simulink model "HW7_v2_simulink"  (R2019b)
settings: Solver=VariableStepAuto  StartTime=0.0  StopTime=15  RelTol=1e-3
values from neighbouring files (symbols this model uses):
  A = double(round(subs(J_x,   [states, inputs], [trim_state, trim_input])*1000)/1000)    [state_decoupling.m]
  A1_wiener = [0 1 ;               0 0]    [HW7_v2_matlab.m]
  Aaileron = A(5:8,5:8)    [state_decoupling.m]
  Aelevator = A(1:4,1:4)    [state_decoupling.m]
  Arudder = A(11:12,11:12)    [state_decoupling.m]
  Athrust = A(9:10,9:10)    [state_decoupling.m]
  B = B*MotorMix    [state_decoupling.m]
  B1_wiener = [0;               1]    [HW7_v2_matlab.m]
  Baileron = B(5:8,3)    [state_decoupling.m]
  Belevator = B(1:4,2)    [state_decoupling.m]
  Brudder = B(11:12,4)    [state_decoupling.m]
  Bthrust = B(9:10,1)    [state_decoupling.m]
  C = double(round(subs(J_y,   [states, inputs], [trim_state, trim_input])*1000)/1000)    [state_decoupling.m]
  C1_wiener = [1 0]    [HW7_v2_matlab.m]
  C_P = 0.041    [state_decoupling.m]
  C_rollpitch = rho*prop_dia^4*prop_dist/sqrt(2)*[                 1  -1  -1   1 ;                 1   1  -1  -1 ;                 0   0   0   0 ; ]    [state_decoupling.m]
  C_T = [0.069075;4.95e-05]    [state_decoupling.m]
  C_yaw = rho*prop_dia^5/(2*pi)*[                 0   0   0   0 ;                 0   0   0   0 ;                -1   1  -1   1 ; ]    [state_decoupling.m]
  Caileron = [0 1 0 0; 0 0 0 1]    [state_decoupling.m]
  Celevator = [0 1 0 0; 0 0 0 1]    [state_decoupling.m]
  Crudder = [0 1]    [state_decoupling.m]
  Cthrust = [ 1 0; 0 0]    [state_decoupling.m]
  D = D*MotorMix    [state_decoupling.m]
  D1_wiener = [0]    [HW7_v2_matlab.m]
  Daileron = [0 ; 0]    [state_decoupling.m]
  Delevator = [0 ; 0]    [state_decoupling.m]
  Drudder = 0    [state_decoupling.m]
  Dthrust = [0 ; D(4,1)]    [state_decoupling.m]
  g = [0;0;UAV_mass*9.81]    [state_decoupling.m]
  J = [      Jxx   0   0 ;       0   Jyy  0 ;       0    0  Jzz; ]    [state_decoupling.m]
  Jinv = inv(J)    [state_decoupling.m]
  Kaileron = Kaileron(2:4)    [HW7_v2_matlab.m]
  Kelevator = Kelevator(2:4)    [HW7_v2_matlab.m]
  Krudder = Krudder(2)    [HW7_v2_matlab.m]
  Kthrust = lqr(Athrust, Bthrust, Qthrust, Rthrust)    [HW7_v2_matlab.m]
  L1 = lqe(A1_cont, G1, C1_cont, Q1, R1, N1)    [HW7_v2_matlab.m]
  M_inv = inv(M_motor)    [HW7_v2_matlab.m]
  M_motor = [1, 1, 1, -1;             1, 1, -1, 1;             1, -1, -1, -1;             1, -1, 1, 1 ]    [HW7_v2_matlab.m]
  Prop_H = 2*pi*Jprop*[               0  0  0  0 ;               0  0  0  0 ;               1 -1  1 -1 ; ]    [state_decoupling.m]
  tau2 = eval(max(solve(1/sqrt((tau2*2*pi*10)^2+1^2) == 1/sqrt(2), tau2)))    [HW7_v2_matlab.m]
  Thrust_Sum = rho*prop_dia^4*[                 0   0   0   0 ;                 0   0   0   0 ;                -1  -1  -1  -1 ; ]    [state_decoupling.m]
  trim_state = [0,0,0,0,0,0,0,0,0,0,0,0]    [state_decoupling.m]
  UAV_mass = 0.068    [state_decoupling.m]
undefined symbols (not defined in the file or in its folder): DiscIntNeverNeededParam, measurement_noise
libraries: simulink x5, vrlib x3, dspmtrx3 x1
settings Model: Creator=cwhipp  LastModifiedBy=cwhipp

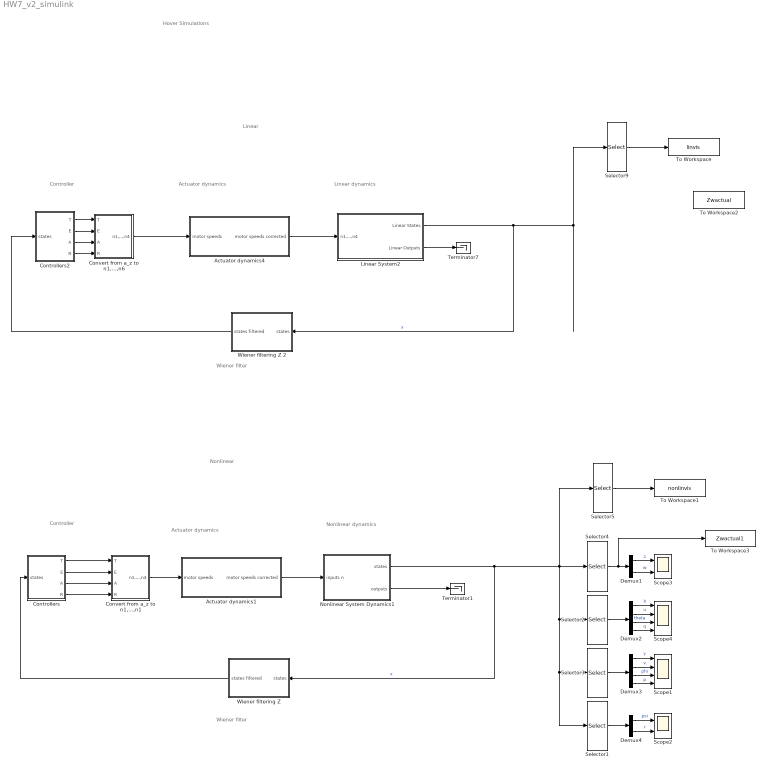
== system HW7_v2_simulink ==
  note: Hover Simulations
  note: Nonlinear
  note: Linear
  note: Controller
  note: Actuator dynamics
  note: Linear dynamics
  note: Wiener filter
  note: Controller
  note: Actuator dynamics
  note: Nonlinear dynamics
  note: Wiener filter
  Actuator dynamics1 : Subsystem
  Actuator dynamics4 : Subsystem
  Controllers : Subsystem
  Controllers2 : Subsystem
  Convert from a_z to n1,...,n1 : Subsystem
  Convert from a_z to n1,...,n6 : Subsystem
  Demux1 : Demux  Outputs=2
  Demux2 : Demux
  Demux3 : Demux
  Demux4 : Demux  Outputs=2
  Linear System2 : Subsystem
  Nonlinear System Dynamics1 : Subsystem
  Scope1 : Scope  NumInputPorts=4
  Scope2 : Scope  NumInputPorts=2
  Scope3 : Scope  NumInputPorts=2
  Scope4 : Scope  NumInputPorts=4
  Selector1 : Selector  InputPortWidth=12  IndexOptions=Index vector (dialog)  Indices=[11 12]  OutputSizes=1
  Selector2 : Selector  InputPortWidth=12  IndexOptions=Index vector (dialog)  Indices=[3 4 5 6]  OutputSizes=1
  Selector3 : Selector  InputPortWidth=12  IndexOptions=Index vector (dialog)  Indices=[7 8 9 10]  OutputSizes=1
  Selector4 : Selector  InputPortWidth=12  IndexOptions=Index vector (dialog)  Indices=[1 2]  OutputSizes=1
  Selector5 : Selector  InputPortWidth=12  IndexOptions=Index vector (dialog)  Indices=[3 7 1 5 9 11]  OutputSizes=1
  Selector9 : Selector  InputPortWidth=12  IndexOptions=Index vector (dialog)  Indices=[3 7 1 5 9 11]  OutputSizes=1
  Terminator1 : Terminator
  Terminator7 : Terminator
  To Workspace : ToWorkspace  VariableName=linvis  SampleTime=-1
      settings: Save2DSignal=2-D array (concatenate along first dimension)
  To Workspace1 : ToWorkspace  VariableName=nonlinvis  SampleTime=-1
      settings: Save2DSignal=2-D array (concatenate along first dimension)
  To Workspace2 : ToWorkspace  VariableName=Zwactual  SaveFormat=Timeseries  SampleTime=-1
  To Workspace3 : ToWorkspace  VariableName=Zwactual1  SaveFormat=Timeseries  SampleTime=-1
  "Wiener filtering Z " : Subsystem
  Wiener filtering Z 2 : Subsystem
  wires:
  Actuator dynamics1/1(motor speeds corrected) -> Nonlinear System Dynamics1/1(inputs n)
  Controllers/4(R) -> Convert from a_z to n1,...,n1/4(R)
  Convert from a_z to n1,...,n1/1(n1,...,n4) -> Actuator dynamics1/1(motor speeds)
  Nonlinear System Dynamics1/2(outputs) -> Terminator1/1
  Controllers/3(A) -> Convert from a_z to n1,...,n1/3(A)
  "Wiener filtering Z "/1("states filtered ") -> Controllers/1(states)
  Controllers/1(T) -> Convert from a_z to n1,...,n1/1(T)
  Controllers/2(E) -> Convert from a_z to n1,...,n1/2(E)
  Actuator dynamics4/1(motor speeds corrected) -> Linear System2/1(n1,...,n4)
  Controllers2/1(T) -> Convert from a_z to n1,...,n6/1(T)
  Convert from a_z to n1,...,n6/1(n1,...,n4) -> Actuator dynamics4/1(motor speeds)
  Controllers2/2(E) -> Convert from a_z to n1,...,n6/2(E)
  Controllers2/4(R) -> Convert from a_z to n1,...,n6/4(R)
  Wiener filtering Z 2/1("states filtered ") -> Controllers2/1(states)
  Controllers2/3(A) -> Convert from a_z to n1,...,n6/3(A)
  Linear System2/2(Linear Outputs) -> Terminator7/1
  Demux4/2 -> Scope2/2  "r"
  Demux3/1 -> Scope1/1  "Y"
  Demux1/1 -> Scope3/1  "z"
  Demux2/4 -> Scope4/4  "q"
  Demux2/3 -> Scope4/3  "theta"
  Demux4/1 -> Scope2/1  "psi"
  Demux2/2 -> Scope4/2  "u"
  Demux1/2 -> Scope3/2  "w"
  Demux3/3 -> Scope1/3  "phi"
  Selector3/1 -> Demux3/1
  Demux2/1 -> Scope4/1  "X"
  Selector1/1 -> Demux4/1
  Selector4/1 -> To Workspace3/1, Demux1/1
  Demux3/4 -> Scope1/4  "p"
  Nonlinear System Dynamics1/1(states) -> Selector5/1, Selector1/1, Selector3/1, Selector2/1, Selector4/1, "Wiener filtering Z "/1(states)  "x"
  Selector2/1 -> Demux2/1
  Demux3/2 -> Scope1/2  "v"
  Selector9/1 -> To Workspace/1
  Linear System2/1(Linear States) -> Selector9/1, Wiener filtering Z 2/1(states)  "x"
  Selector5/1 -> To Workspace1/1

== system HW7_v2_simulink/Actuator dynamics1 ==
  motor speeds : Inport
  30ms delay : TransportDelay  DelayTime=30e-3
  Demux : Demux
  Mux : Mux
  Saturation4 : Saturate  UpperLimit=500  LowerLimit=10
  Sum2 : Sum  Inputs=++|
  Transfer Fcn : TransferFcn  Denominator=[tau2 1]
  Transfer Fcn1 : TransferFcn  Denominator=[tau2 1]
  Transfer Fcn2 : TransferFcn  Denominator=[tau2 1]
  actuator transfer function : TransferFcn  Denominator=[tau2 1]
  speed correction : Constant  Value=293
  motor speeds corrected : Outport
  wires:
  speed correction/1 -> Sum2/1
  Sum2/1 -> Saturation4/1
  Demux/2 -> Transfer Fcn1/1
  30ms delay/1 -> Demux/1
  Demux/4 -> actuator transfer function/1
  Demux/1 -> Transfer Fcn/1
  Demux/3 -> Transfer Fcn2/1
  Transfer Fcn/1 -> Mux/1
  Transfer Fcn1/1 -> Mux/2
  Transfer Fcn2/1 -> Mux/3
  actuator transfer function/1 -> Mux/4
  Mux/1 -> Sum2/2
  Saturation4/1 -> motor speeds corrected/1
  motor speeds/1 -> 30ms delay/1

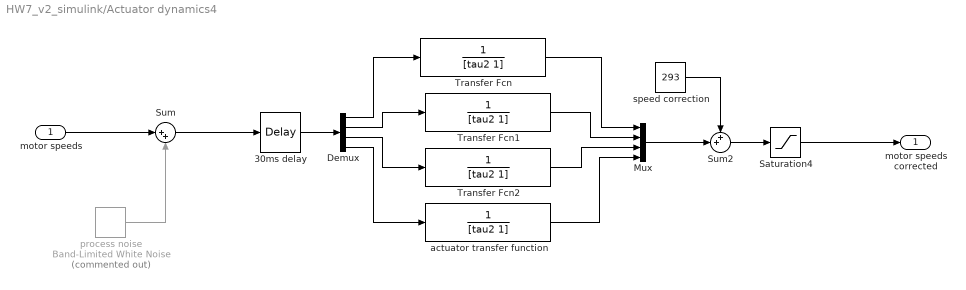
== system HW7_v2_simulink/Actuator dynamics4 ==
  motor speeds : Inport
  30ms delay : TransportDelay  DelayTime=30e-3
  Demux : Demux
  Mux : Mux
  Saturation4 : Saturate  UpperLimit=500  LowerLimit=10
  Sum : Sum  Inputs=|++
  Sum2 : Sum  Inputs=++|
  Transfer Fcn : TransferFcn  Denominator=[tau2 1]
  Transfer Fcn1 : TransferFcn  Denominator=[tau2 1]
  Transfer Fcn2 : TransferFcn  Denominator=[tau2 1]
  actuator transfer function : TransferFcn  Denominator=[tau2 1]
  process noise : simulink/Sources/Band-Limited White Noise  Commented=on  Cov=0.005*[1; 1; 1; 1]  Ts=0.005  seed=[1; 2; 3; 4]
  speed correction : Constant  Value=293  SampleTime=0.005
  motor speeds corrected : Outport
  wires:
  speed correction/1 -> Sum2/1
  Sum2/1 -> Saturation4/1
  Demux/2 -> Transfer Fcn1/1
  30ms delay/1 -> Demux/1
  Demux/4 -> actuator transfer function/1
  Demux/1 -> Transfer Fcn/1
  Demux/3 -> Transfer Fcn2/1
  Transfer Fcn/1 -> Mux/1
  Transfer Fcn1/1 -> Mux/2
  Transfer Fcn2/1 -> Mux/3
  actuator transfer function/1 -> Mux/4
  Mux/1 -> Sum2/2
  Saturation4/1 -> motor speeds corrected/1
  process noise/1 -> Sum/2
  motor speeds/1 -> Sum/1
  Sum/1 -> 30ms delay/1

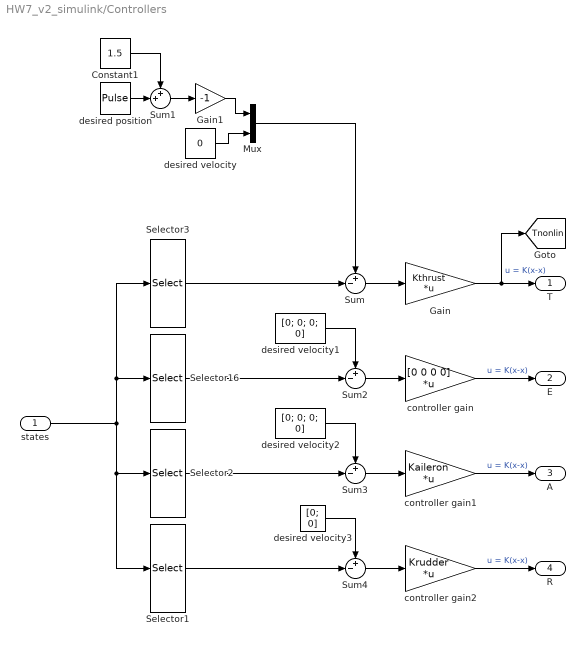
== system HW7_v2_simulink/Controllers ==
  states : Inport
  Constant1 : Constant  Value=1.5  SampleTime=0.05
  Gain : Gain  Gain=Kthrust  Multiplication=Matrix(K*u)
  Gain1 : Gain  Gain=-1
  Mux : Mux  Inputs=2
  Selector1 : Selector  InputPortWidth=12  IndexOptions=Index vector (dialog)  Indices=[11 12]  OutputSizes=1
  Selector16 : Selector  InputPortWidth=12  IndexOptions=Index vector (dialog)  Indices=[3 4 5 6]  OutputSizes=1
  Selector2 : Selector  InputPortWidth=12  IndexOptions=Index vector (dialog)  Indices=[7 8 9 10]  OutputSizes=1
  Selector3 : Selector  InputPortWidth=12  IndexOptions=Index vector (dialog)  Indices=[1 2]  OutputSizes=1
  Sum{,2..4} (4 alike) : Sum  Inputs=+-|
  Sum1 : Sum  Inputs=++|
  controller gain : Gain  Gain=[0 0 0 0]  Multiplication=Matrix(K*u)
  controller gain1 : Gain  Gain=Kaileron  Multiplication=Matrix(K*u)
  controller gain2 : Gain  Gain=Krudder  Multiplication=Matrix(K*u)
  desired position : DiscretePulseGenerator  PulseType=Time based  Amplitude=-1.5  Period=10  PulseWidth=50
  desired velocity : Constant  Value=0  SampleTime=0.05
  desired velocity1 : Constant  Value=[0; 0; 0; 0]  SampleTime=0.05
  desired velocity2 : Constant  Value=[0; 0; 0; 0]  SampleTime=0.05
  desired velocity3 : Constant  Value=[0; 0]  SampleTime=0.05
  T : Outport
  E : Outport  Port=2
  A : Outport  Port=3
  R : Outport  Port=4
  tag scope: Tnonlin=global
  wires:
  states/1 -> Selector16/1, Selector3/1, Selector1/1, Selector2/1
  Mux/1 -> Sum/1
  Gain1/1 -> Mux/1
  Sum/1 -> Gain/1
  Sum1/1 -> Gain1/1
  Selector3/1 -> Sum/2
  Constant1/1 -> Sum1/1
  Gain/1 -> [Tnonlin], T/1  "u = K(x-x)"
  desired position/1 -> Sum1/2
  Selector16/1 -> Sum2/2
  desired velocity1/1 -> Sum2/1
  Sum2/1 -> controller gain/1
  controller gain/1 -> E/1  "u = K(x-x)"
  Selector2/1 -> Sum3/2
  controller gain1/1 -> A/1  "u = K(x-x)"
  desired velocity2/1 -> Sum3/1
  Sum3/1 -> controller gain1/1
  controller gain2/1 -> R/1  "u = K(x-x)"
  Sum4/1 -> controller gain2/1
  desired velocity3/1 -> Sum4/1
  Selector1/1 -> Sum4/2
  desired velocity/1 -> Mux/2

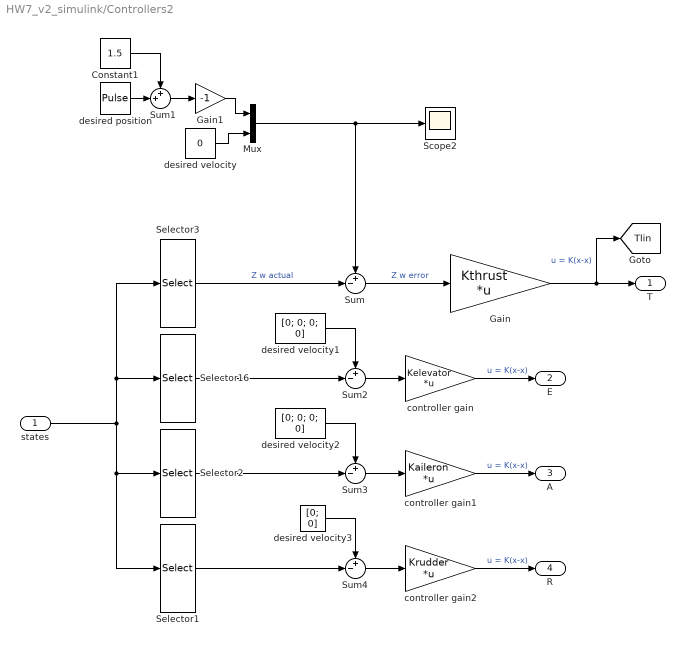
== system HW7_v2_simulink/Controllers2 ==
  states : Inport
  Constant1 : Constant  Value=1.5  SampleTime=0.05
  Gain : Gain  Gain=Kthrust  Multiplication=Matrix(K*u)
  Gain1 : Gain  Gain=-1
  Mux : Mux  Inputs=2
  Scope2 : Scope
  Selector1 : Selector  InputPortWidth=12  IndexOptions=Index vector (dialog)  Indices=[11 12]  OutputSizes=1
  Selector16 : Selector  InputPortWidth=12  IndexOptions=Index vector (dialog)  Indices=[3 4 5 6]  OutputSizes=1
  Selector2 : Selector  InputPortWidth=12  IndexOptions=Index vector (dialog)  Indices=[7 8 9 10]  OutputSizes=1
  Selector3 : Selector  InputPortWidth=12  IndexOptions=Index vector (dialog)  Indices=[1 2]  OutputSizes=1
  Sum{,2..4} (4 alike) : Sum  Inputs=+-|
  Sum1 : Sum  Inputs=++|
  controller gain : Gain  Gain=Kelevator  Multiplication=Matrix(K*u)
  controller gain1 : Gain  Gain=Kaileron  Multiplication=Matrix(K*u)
  controller gain2 : Gain  Gain=Krudder  Multiplication=Matrix(K*u)
  desired position : DiscretePulseGenerator  PulseType=Time based  Amplitude=-1.5  Period=10  PulseWidth=50
  desired velocity : Constant  Value=0  SampleTime=0.05
  desired velocity1 : Constant  Value=[0; 0; 0; 0]  SampleTime=0.05
  desired velocity2 : Constant  Value=[0; 0; 0; 0]  SampleTime=0.05
  desired velocity3 : Constant  Value=[0; 0]  SampleTime=0.05
  T : Outport
  E : Outport  Port=2
  A : Outport  Port=3
  R : Outport  Port=4
  tag scope: Tlin=global
  wires:
  states/1 -> Selector16/1, Selector3/1, Selector2/1, Selector1/1
  Mux/1 -> Scope2/1, Sum/1
  Gain1/1 -> Mux/1
  Sum/1 -> Gain/1  "Z w error"
  Sum1/1 -> Gain1/1
  Constant1/1 -> Sum1/1
  Gain/1 -> T/1, [Tlin]  "u = K(x-x)"
  desired position/1 -> Sum1/2
  desired velocity1/1 -> Sum2/1
  Sum2/1 -> controller gain/1
  controller gain/1 -> E/1  "u = K(x-x)"
  controller gain1/1 -> A/1  "u = K(x-x)"
  desired velocity2/1 -> Sum3/1
  Sum3/1 -> controller gain1/1
  controller gain2/1 -> R/1  "u = K(x-x)"
  Sum4/1 -> controller gain2/1
  desired velocity3/1 -> Sum4/1
  desired velocity/1 -> Mux/2
  Selector3/1 -> Sum/2  "Z w actual"
  Selector16/1 -> Sum2/2
  Selector2/1 -> Sum3/2
  Selector1/1 -> Sum4/2

== system HW7_v2_simulink/Convert from a_z to n1,...,n1 ==
  T : Inport
  E : Inport  Port=2
  A : Inport  Port=3
  R : Inport  Port=4
  Convert fom TEAR to n1,..,n4 : Gain  Gain=M_motor  Multiplication=Matrix(K*u)
  Mux : Mux
  n1,...,n4 : Outport
  wires:
  Convert fom TEAR to n1,..,n4/1 -> n1,...,n4/1
  Mux/1 -> Convert fom TEAR to n1,..,n4/1
  T/1 -> Mux/1
  E/1 -> Mux/2
  A/1 -> Mux/3
  R/1 -> Mux/4

== system HW7_v2_simulink/Convert from a_z to n1,...,n6 ==
  T : Inport
  E : Inport  Port=2
  A : Inport  Port=3
  R : Inport  Port=4
  Convert fom TEAR to n1,..,n4 : Gain  Gain=M_motor  Multiplication=Matrix(K*u)
  Mux : Mux
  n1,...,n4 : Outport
  wires:
  Convert fom TEAR to n1,..,n4/1 -> n1,...,n4/1
  Mux/1 -> Convert fom TEAR to n1,..,n4/1
  T/1 -> Mux/1
  E/1 -> Mux/2
  A/1 -> Mux/3
  R/1 -> Mux/4

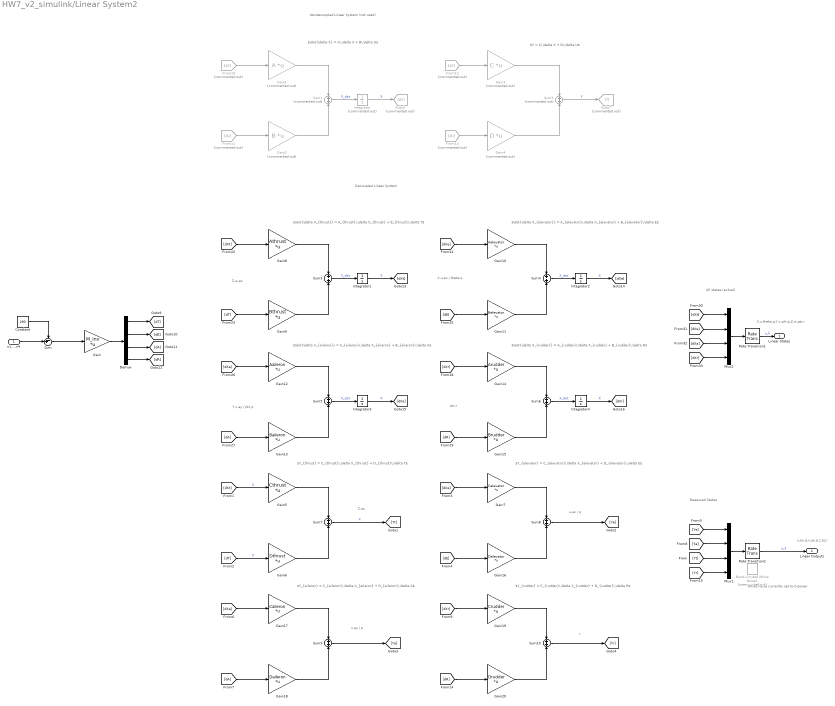
== system HW7_v2_simulink/Linear System2 ==
  note: psi,r
  note: Y,v,ay / phi,p
  note: X,u,ax / theta,q
  note: Z,w,az
  note: Decoupled Linear System
  note: $\dot{\delta X} = A\,\delta X + B\,\delta U$
  note: $Y = C\,\delta X + D\,\delta U$
  note: $\dot{\delta X_{thrust}} = A_{thrust}\,\delta X_{thrust} + B_{thrust}\,\delta T$
  note: $\dot{\delta X_{elevator}} = A_{elevator}\,\delta X_{elevator} + B_{elevator}\,\delta E$
  note: $\dot{\delta X_{aileron}} = A_{aileron}\,\delta X_{aileron} + B_{aileron}\,\delta A$
  note: $\dot{\delta X_{rudder}} = A_{rudder}\,\delta X_{rudder} + B_{rudder}\,\delta R$
  note: Z,az
  note: u,ax / q
  note: v,ay / p
  note: r
  note: $Y_{thrust} = C_{thrust}\,\delta X_{thrust} + D_{thrust}\,\delta T$
  note: $Y_{elevator} = C_{elevator}\,\delta X_{elevator} + D_{elevator}\,\delta E$
  note: $Y_{aileron} = C_{aileron}\,\delta X_{aileron} + D_{aileron}\,\delta A$
  note: $Y_{rudder} = C_{rudder}\,\delta X_{rudder} + D_{rudder}\,\delta R$
  note: Nondecoupled Linear System (not used)
  note: All states (actual)
  note: Measured States
  note: u,ax,q,v,ay,p,z,az,r
  note: X,u,theta,q,Y,v,phi,p,Z,w,psi,r
  note: White noise currently set to 0 power
  n1,...,n4 : Inport
  Band-Limited White Noise1 : simulink/Sources/Band-Limited White Noise  Commented=on  Cov=measurement_noise*ones(9,1)*0  Ts=0.05  seed=[11;12;13;14;15;16;17;18;19]
  Constant : Constant  Value=293
  Demux : Demux
  From10 : From  Commented=on  GotoTag=dX
  From11 : From  Commented=on  GotoTag=dU
  From12 : From  Commented=on  GotoTag=dX
  From13 : From  Commented=on  GotoTag=dU
  Gain : Gain  Gain=M_inv  Multiplication=Matrix(K*u)
  Gain1 : Gain  Commented=on  Gain=A  Multiplication=Matrix(K*u)
  Gain10 : Gain  Gain=Aelevator  Multiplication=Matrix(K*u)
  Gain11 : Gain  Gain=Belevator  Multiplication=Matrix(K*u)
  Gain12 : Gain  Gain=Aaileron  Multiplication=Matrix(K*u)
  Gain13 : Gain  Gain=Baileron  Multiplication=Matrix(K*u)
  Gain14 : Gain  Gain=Arudder  Multiplication=Matrix(K*u)
  Gain15 : Gain  Gain=Brudder  Multiplication=Matrix(K*u)
  Gain16 : Gain  Gain=Delevator  Multiplication=Matrix(K*u)
  Gain17 : Gain  Gain=Caileron  Multiplication=Matrix(K*u)
  Gain18 : Gain  Gain=Daileron  Multiplication=Matrix(K*u)
  Gain19 : Gain  Gain=Crudder  Multiplication=Matrix(K*u)
  Gain2 : Gain  Commented=on  Gain=B  Multiplication=Matrix(K*u)
  Gain20 : Gain  Gain=Drudder  Multiplication=Matrix(K*u)
  Gain3 : Gain  Commented=on  Gain=C  Multiplication=Matrix(K*u)
  Gain4 : Gain  Commented=on  Gain=D  Multiplication=Matrix(K*u)
  Gain5 : Gain  Gain=Cthrust  Multiplication=Matrix(K*u)
  Gain6 : Gain  Gain=Dthrust  Multiplication=Matrix(K*u)
  Gain7 : Gain  Gain=Celevator  Multiplication=Matrix(K*u)
  Gain8 : Gain  Gain=Athrust  Multiplication=Matrix(K*u)
  Gain9 : Gain  Gain=Bthrust  Multiplication=Matrix(K*u)
  Goto5 : Goto  Commented=on  GotoTag=dX
  Goto7 : Goto  Commented=on  GotoTag=Y
  Integrator : Integrator  Commented=on  InitialCondition=trim_state
  Integrator1 : Integrator  InitialCondition=trim_state(9:10)
  Integrator2 : Integrator  InitialCondition=trim_state(1:4)
  Integrator3 : Integrator  InitialCondition=trim_state(5:8)
  Integrator4 : Integrator  InitialCondition=trim_state(11:12)
  Mux1 : Mux
  Mux2 : Mux
  Rate Transition1 : RateTransition  OutPortSampleTime=0.005
  Rate Transition2 : RateTransition  OutPortSampleTime=0.005
  Sum : Sum  Inputs=-+|
  Sum1 : Sum  Commented=on  Inputs=+|+
  Sum{3..10} (8 alike) : Sum  Inputs=+|+
  Sum2 : Sum  Commented=on  Inputs=+|+
  Linear States : Outport
  Linear Outputs : Outport  Port=2
  wires:
  Gain14/1 -> Sum6/1
  From11/1 -> Gain2/1
  [dXe] -> Gain10/1
  Gain10/1 -> Sum4/1
  Gain2/1 -> Sum1/2
  Gain15/1 -> Sum6/2
  Gain1/1 -> Sum1/1
  Sum5/1 -> Integrator3/1  "X_dot"
  Gain3/1 -> Sum2/1
  Integrator1/1 -> [dXt]  "X"
  From10/1 -> Gain1/1
  Sum1/1 -> Integrator/1  "X_dot"
  Sum2/1 -> Goto7/1  "Y"
  Integrator3/1 -> [dXa]  "X"
  Gain8/1 -> Sum3/1
  [dXt] -> Gain8/1
  Sum3/1 -> Integrator1/1  "X_dot"
  Integrator4/1 -> [dXr]  "X"
  Sum4/1 -> Integrator2/1  "X_dot"
  Gain13/1 -> Sum5/2
  [dXa] -> Gain12/1
  [dXr] -> Gain14/1
  Sum6/1 -> Integrator4/1  "X_dot"
  From13/1 -> Gain4/1
  Gain11/1 -> Sum4/2
  Integrator/1 -> Goto5/1  "X"
  Gain4/1 -> Sum2/2
  Gain12/1 -> Sum5/1
  Integrator2/1 -> [dXe]  "X"
  From12/1 -> Gain3/1
  Gain/1 -> Demux/1
  Demux/3 -> [dA]
  Demux/2 -> [dE]
  Demux/1 -> [dT]
  Demux/4 -> [dR]
  [dXa] -> Mux2/3
  [dXr] -> Mux2/4
  Mux2/1 -> Rate Transition1/1
  [dXt] -> Mux2/1
  [dXe] -> Mux2/2
  Gain6/1 -> Sum7/2
  Gain5/1 -> Sum7/1
  Gain16/1 -> Sum8/2
  [dE] -> Gain16/1
  Gain7/1 -> Sum8/1
  [dXe] -> Gain7/1
  [dA] -> Gain18/1
  Gain17/1 -> Sum9/1
  [dXa] -> Gain17/1
  Gain18/1 -> Sum9/2
  [dXr] -> Gain19/1
  [dR] -> Gain20/1
  Gain20/1 -> Sum10/2
  Gain19/1 -> Sum10/1
  [Ya] -> Mux1/2
  [Ye] -> Mux1/1
  Mux1/1 -> Rate Transition2/1
  [Yr] -> Mux1/4
  [Yt] -> Mux1/3
  [dT] -> Gain9/1
  [dA] -> Gain13/1
  [dR] -> Gain15/1
  [dE] -> Gain11/1
  Sum9/1 -> [Ya]
  Sum10/1 -> [Yr]
  Sum8/1 -> [Ye]
  Gain9/1 -> Sum3/2
  [dT] -> Gain6/1  "X"
  [dXt] -> Gain5/1  "X"
  Sum7/1 -> [Yt]  "X"
  Rate Transition1/1 -> Linear States/1  "x_k"
  Rate Transition2/1 -> Linear Outputs/1  "y_k"
  n1,...,n4/1 -> Sum/2
  Constant/1 -> Sum/1
  Sum/1 -> Gain/1

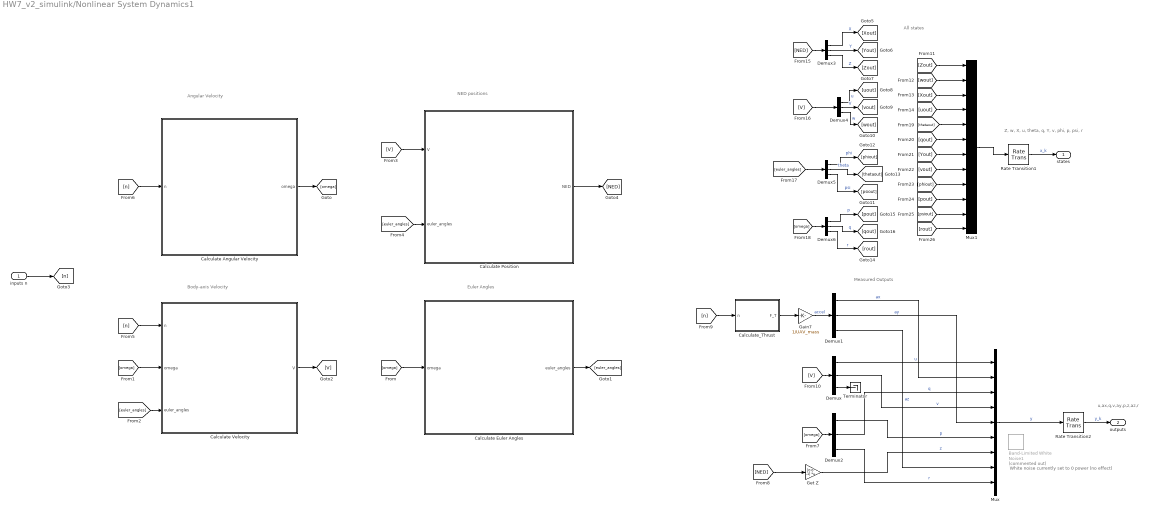
== system HW7_v2_simulink/Nonlinear System Dynamics1 ==
  note: White noise currently set to 0 power (no effect)
  note: Z, w, X, u, theta, q, Y, v, phi, p, psi, r
  note: Euler Angles
  note: NED positions
  note: Angular Velocity
  note: Body-axis Velocity
  note: u,ax,q,v,ay,p,z,az,r
  note: All states
  note: Measured Outputs
  inputs n : Inport
  Band-Limited White Noise1 : simulink/Sources/Band-Limited White Noise  Commented=on  Cov=measurement_noise*ones(9,1)*0  Ts=0.05  seed=[11;12;13;14;15;16;17;18;19]
  Calculate Angular Velocity : Subsystem
  Calculate Euler Angles : Subsystem
  Calculate Position : Subsystem
  Calculate Velocity : Subsystem
  Calculate_Thrust : Subsystem
  Demux{,1..6} (7 alike) : Demux  Outputs=3
  Gain7 : Gain  Gain=1/UAV_mass
      settings: AttributesFormatString=%<Gain>
  Get Z : Gain  Gain=[0 0 -1]  Multiplication=Matrix(K*u)
  Mux : Mux  Inputs=9
  Mux1 : Mux  Inputs=12
  Rate Transition1 : RateTransition  OutPortSampleTime=0.005
  Rate Transition2 : RateTransition  OutPortSampleTime=0.005
  Terminator : Terminator
  states : Outport
  outputs : Outport  Port=2
  wires:
  [euler_angles] -> Demux5/1
  [omega] -> Demux6/1
  Calculate Euler Angles/1(euler_angles) -> [euler_angles]
  [V] -> Calculate Position/1("V ")
  [euler_angles] -> Calculate Position/2(euler_angles)
  Calculate Angular Velocity/1(omega) -> [omega]
  [omega] -> Calculate Euler Angles/1(omega)
  Calculate Velocity/1(V) -> [V]
  [V] -> Demux4/1
  [NED] -> Demux3/1
  [euler_angles] -> Calculate Velocity/3(euler_angles)
  [omega] -> Calculate Velocity/2(omega)
  [n] -> Calculate Velocity/1(n)
  Calculate Position/1(NED) -> [NED]
  [n] -> Calculate Angular Velocity/1(n)
  inputs n/1 -> [n]
  Demux1/1 -> Mux/2  "ax"
  Demux/1 -> Mux/1  "u"
  Mux/1 -> Rate Transition2/1  "y"
  Demux/3 -> Terminator/1
  [omega] -> Demux2/1
  [NED] -> Get Z/1
  Get Z/1 -> Mux/7  "z"
  Demux2/2 -> Mux/3  "q"
  Demux/2 -> Mux/4  "v"
  Demux2/1 -> Mux/6  "p"
  Demux1/2 -> Mux/5  "ay"
  Demux2/3 -> Mux/9  "r"
  [V] -> Demux/1
  Demux1/3 -> Mux/8  "az"
  Gain7/1 -> Demux1/1  "accel"
  Calculate_Thrust/1(F_T) -> Gain7/1
  [n] -> Calculate_Thrust/1(n)
  Rate Transition1/1 -> states/1  "x_k"
  Rate Transition2/1 -> outputs/1  "y_k"
  Mux1/1 -> Rate Transition1/1
  Demux3/1 -> [Xout]  "X"
  Demux3/2 -> [Yout]  "Y"
  Demux3/3 -> [Zout]  "Z"
  Demux4/1 -> [uout]  "u"
  Demux4/2 -> [vout]  "V"
  Demux4/3 -> [wout]  "w"
  Demux5/1 -> [phiout]  "phi"
  Demux5/2 -> [thetaout]  "theta"
  Demux5/3 -> [psiout]  "psi"
  Demux6/1 -> [pout]  "p"
  Demux6/2 -> [qout]  "q"
  Demux6/3 -> [rout]  "r"
  [Zout] -> Mux1/1
  [wout] -> Mux1/2
  [rout] -> Mux1/12
  [psiout] -> Mux1/11
  [pout] -> Mux1/10
  [phiout] -> Mux1/9
  [vout] -> Mux1/8
  [Yout] -> Mux1/7
  [qout] -> Mux1/6
  [uout] -> Mux1/4
  [Xout] -> Mux1/3
  [thetaout] -> Mux1/5

== system HW7_v2_simulink/Wiener filtering Z  ==
  states : Inport
  Demux : Demux  Outputs=2
  Gain5 : Gain  Gain=-0.067
  Mux : Mux  Inputs=5
  ZNED : Selector  InputPortWidth=12  IndexOptions=Index vector (dialog)  Indices=[3]  OutputSizes=1
  states 1 2 : Selector  InputPortWidth=12  IndexOptions=Index vector (dialog)  Indices=[1 2]  OutputSizes=1
  "states 4, 5" : Selector  InputPortWidth=12  IndexOptions=Index vector (dialog)  Indices=[4 5]  OutputSizes=1
  states 7-12 : Selector  InputPortWidth=12  IndexOptions=Index vector (dialog)  Indices=[7 8 9 10 11 12]  OutputSizes=1
  zw wiener filter2 : Subsystem
  "states filtered " : Outport
  wires:
  "states 4, 5"/1 -> Mux/3
  states 1 2/1 -> Mux/1
  states/1 -> states 7-12/1, "states 4, 5"/1, ZNED/1, states 1 2/1
  ZNED/1 -> zw wiener filter2/2(z)
  Gain5/1 -> zw wiener filter2/1(az)  "wdot = a_z"
  [Tnonlin] -> Gain5/1
  Mux/1 -> "states filtered "/1
  zw wiener filter2/1(zw_wiener) -> Demux/1  "zw"
  Demux/1 -> Mux/2
  Demux/2 -> Mux/4
  states 7-12/1 -> Mux/5

== system HW7_v2_simulink/Wiener filtering Z 2 ==
  states : Inport
  Gain5 : Gain  Gain=-0.067
  Mux : Mux  Inputs=2
  ZNED : Selector  InputPortWidth=12  IndexOptions=Index vector (dialog)  Indices=[1]  OutputSizes=1
  Zw Wiener filter : Subsystem
  states 3-12 : Selector  InputPortWidth=12  IndexOptions=Index vector (dialog)  Indices=[3 4 5 6 7 8 9 10 11 12]  OutputSizes=1
  "states filtered " : Outport
  wires:
  states/1 -> states 3-12/1, ZNED/1
  ZNED/1 -> Zw Wiener filter/2(z)
  Gain5/1 -> Zw Wiener filter/1(az)  "wdot = a_z"
  [Tlin] -> Gain5/1
  Mux/1 -> "states filtered "/1
  Zw Wiener filter/1(zw_wiener) -> Mux/1  "zw"
  states 3-12/1 -> Mux/2

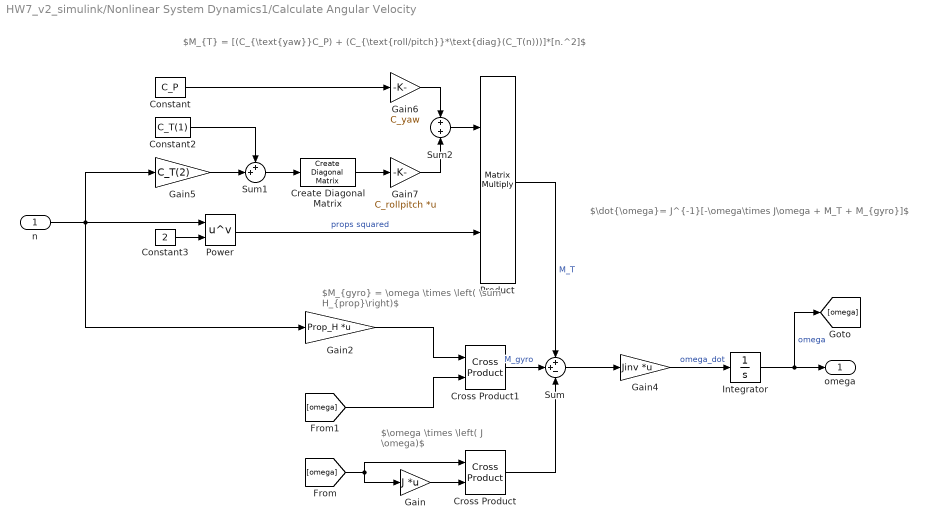
== system HW7_v2_simulink/Nonlinear System Dynamics1/Calculate Angular Velocity ==
  note: $M_{gyro} = \omega \times \left( \sum H_{prop}\right)$
  note: $\dot{\omega}= J^{-1}[-\omega\times J\omega + M_T + M_{gyro}]$
  note: $\omega \times \left( J \omega)$
  note: $M_{T} = [(C_{\text{yaw}}C_P) + (C_{\text{roll/pitch}}*\text{diag}(C_T(n)))]*[n.^2]$
  n : Inport
  Constant : Constant  Value=C_P
  Constant2 : Constant  Value=C_T(1)
  Constant3 : Constant  Value=2
  Create Diagonal Matrix : dspmtrx3/Create Diagonal Matrix
      settings: SourceProductName=DSP System Toolbox  SourceProductBaseCode=DS
  Cross Product : vrlib/Utilities/Cross Product
      settings: SourceProductName=Simulink
  Cross Product1 : vrlib/Utilities/Cross Product
      settings: SourceProductName=Simulink
  Gain : Gain  Gain=J  Multiplication=Matrix(K*u)
  Gain2 : Gain  Gain=Prop_H  Multiplication=Matrix(K*u)
  Gain4 : Gain  Gain=Jinv  Multiplication=Matrix(K*u)
      settings: AttributesFormatString=%<Gain>
  Gain5 : Gain  Gain=C_T(2)
  Gain6 : Gain  Gain=C_yaw
      settings: AttributesFormatString=%<Gain>
  Gain7 : Gain  Gain=C_rollpitch  Multiplication=Matrix(K*u)
      settings: AttributesFormatString=%<Gain>
  Integrator : Integrator  InitialCondition=[0;0;0]
  Power : Math  Operator=pow  SignedPower=off  SaturateOnIntegerOverflow=on
  Product : Product  Multiplication=Matrix(*)
  Sum : Sum  Inputs=++-
  Sum1 : Sum  Inputs=++|
  Sum2 : Sum  Inputs=+|+
  omega : Outport
  wires:
  Sum/1 -> Gain4/1
  [omega] -> Gain/1, Cross Product/1
  Cross Product/1 -> Sum/3
  [omega] -> Cross Product1/2
  Gain2/1 -> Cross Product1/1
  Cross Product1/1 -> Sum/2  "M_gyro"
  Gain4/1 -> Integrator/1  "omega_dot"
  Gain/1 -> Cross Product/2
  Integrator/1 -> [omega], omega/1  "omega"
  Product/1 -> Sum/1  "M_T"
  Create Diagonal Matrix/1 -> Gain7/1
  Sum2/1 -> Product/1
  Sum1/1 -> Create Diagonal Matrix/1
  Constant/1 -> Gain6/1
  Power/1 -> Product/2  "props squared"
  Gain6/1 -> Sum2/1
  Gain5/1 -> Sum1/2
  Gain7/1 -> Sum2/2
  n/1 -> Gain2/1, Power/1, Gain5/1
  Constant2/1 -> Sum1/1
  Constant3/1 -> Power/2

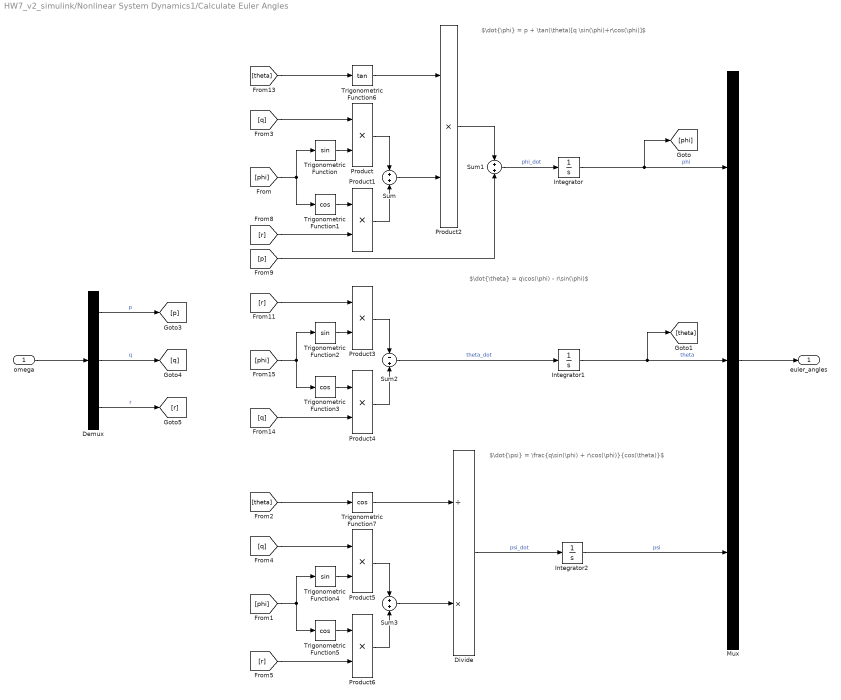
== system HW7_v2_simulink/Nonlinear System Dynamics1/Calculate Euler Angles ==
  note: $\dot{\phi} = p + \tan(\theta)[q \sin(\phi)+r\cos(\phi)]$
  note: $\dot{\theta} = q\cos(\phi) - r\sin(\phi)$
  note: $\dot{\psi} = \frac{q\sin(\phi) + r\cos(\phi)}{cos(\theta)}$
  omega : Inport
  Demux : Demux  Outputs=3
  Divide : Product  Inputs=/*
  Integrator : Integrator
  Integrator1 : Integrator
  Integrator2 : Integrator
  Mux : Mux  Inputs=3
  Product{,1..6} (7 alike) : Product
  Sum : Sum  Inputs=+|+
  Sum1 : Sum  Inputs=+|+
  Sum2 : Sum  Inputs=-|+
  Sum3 : Sum  Inputs=+|+
  Trigonometric Function : Trigonometry
  Trigonometric Function{1,3,5,7} (4 alike) : Trigonometry  Operator=cos
  Trigonometric Function2 : Trigonometry
  Trigonometric Function4 : Trigonometry
  Trigonometric Function6 : Trigonometry  Operator=tan
  euler_angles : Outport
  wires:
  Trigonometric Function7/1 -> Divide/1
  Product1/1 -> Sum/2
  Product6/1 -> Sum3/2
  Trigonometric Function/1 -> Product/2
  Product5/1 -> Sum3/1
  [theta] -> Trigonometric Function7/1
  Trigonometric Function6/1 -> Product2/1
  [r] -> Product6/2
  [theta] -> Trigonometric Function6/1
  Integrator1/1 -> [theta], Mux/2  "theta"
  Trigonometric Function4/1 -> Product5/2
  [q] -> Product4/2
  Demux/3 -> [r]  "r"
  Divide/1 -> Integrator2/1  "psi_dot"
  Integrator2/1 -> Mux/3  "psi"
  [q] -> Product5/1
  Product4/1 -> Sum2/2
  [q] -> Product/1
  [phi] -> Trigonometric Function4/1, Trigonometric Function5/1
  Sum2/1 -> Integrator1/1  "theta_dot"
  Trigonometric Function5/1 -> Product6/1
  Trigonometric Function3/1 -> Product4/1
  [r] -> Product3/1
  Integrator/1 -> [phi], Mux/1  "phi"
  Sum3/1 -> Divide/2
  Product3/1 -> Sum2/1
  [phi] -> Trigonometric Function2/1, Trigonometric Function3/1
  Demux/1 -> [p]  "p"
  Product2/1 -> Sum1/1
  [r] -> Product1/2
  Trigonometric Function1/1 -> Product1/1
  [phi] -> Trigonometric Function1/1, Trigonometric Function/1
  omega/1 -> Demux/1
  Product/1 -> Sum/1
  Demux/2 -> [q]  "q"
  Sum/1 -> Product2/2
  Mux/1 -> euler_angles/1
  Sum1/1 -> Integrator/1  "phi_dot"
  [p] -> Sum1/2
  Trigonometric Function2/1 -> Product3/2

== system HW7_v2_simulink/Nonlinear System Dynamics1/Calculate Position ==
  note: $R(\phi,\theta,\psi)^{-1} = [R(\psi) R(\theta) R(\psi)]^T$
  note: $\dot{NED} = R(\phi,\theta,\psi)^{-1}V$
  "V " : Inport
  euler_angles : Inport  Port=2
  Integrator : Integrator  InitialCondition=[0;0;0]
  Product2 : Product  Multiplication=Matrix(*)
  Rotation_Matrix : Subsystem
  Transpose : Math  Operator=transpose  SignedPower=off  SaturateOnIntegerOverflow=on
  NED : Outport
  wires:
  Product2/1 -> Integrator/1  "NED_dot"
  "V "/1 -> [V]
  Rotation_Matrix/1(Rotation_Matrix) -> Transpose/1  "Rotation_Matrix"
  Transpose/1 -> Product2/1  "Inverse_Rotation_Matrix"
  [V] -> Product2/2
  euler_angles/1 -> Rotation_Matrix/1("euler_angles ")
  Integrator/1 -> NED/1

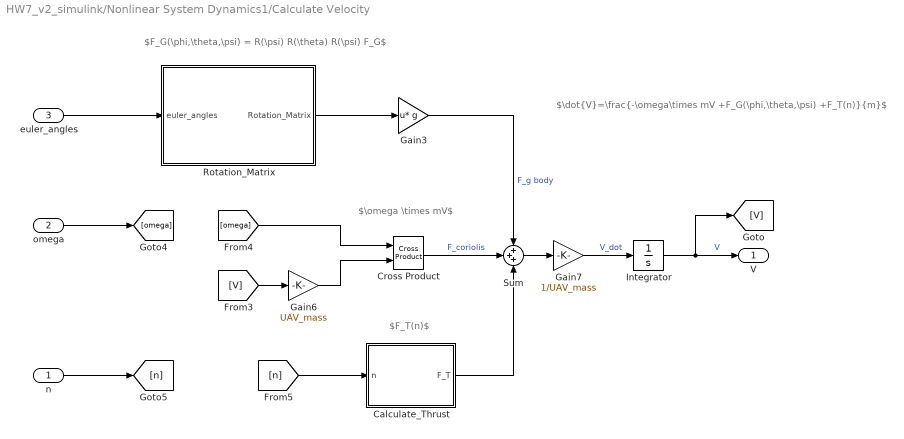
== system HW7_v2_simulink/Nonlinear System Dynamics1/Calculate Velocity ==
  note: $F_G(\phi,\theta,\psi) = R(\psi) R(\theta) R(\psi) F_G$
  note: $\dot{V}=\frac{-\omega\times mV +F_G(\phi,\theta,\psi) +F_T(n)}{m}$
  note: $\omega \times mV$
  note: $F_T(n)$
  n : Inport
  omega : Inport  Port=2
  euler_angles : Inport  Port=3
  Calculate_Thrust : Subsystem
  Cross Product : vrlib/Utilities/Cross Product
      settings: SourceProductName=Simulink
  Gain3 : Gain  Gain=g  Multiplication=Matrix(u*K)
      settings: AttributesFormatString=%<Gain>
  Gain6 : Gain  Gain=UAV_mass
      settings: AttributesFormatString=%<Gain>
  Gain7 : Gain  Gain=1/UAV_mass
      settings: AttributesFormatString=%<Gain>
  Integrator : Integrator  InitialCondition=[0;0;0]
  Rotation_Matrix : Subsystem
  Sum : Sum  Inputs=+++
  V : Outport
  wires:
  [V] -> Gain6/1
  [omega] -> Cross Product/1
  Cross Product/1 -> Sum/2  "F_coriolis"
  Gain3/1 -> Sum/1  "F_g body"
  Gain6/1 -> Cross Product/2
  Sum/1 -> Gain7/1
  Integrator/1 -> V/1, [V]  "V"
  omega/1 -> [omega]
  n/1 -> [n]
  Rotation_Matrix/1(Rotation_Matrix) -> Gain3/1
  euler_angles/1 -> Rotation_Matrix/1("euler_angles ")
  [n] -> Calculate_Thrust/1(n)
  Gain7/1 -> Integrator/1  "V_dot"
  Calculate_Thrust/1(F_T) -> Sum/3

== system HW7_v2_simulink/Nonlinear System Dynamics1/Calculate_Thrust ==
  note: $F_{T} = \sum_{i=1}^4[0;0;C_{T}.*n.^2]$
  n : Inport
  Constant15 : Constant  Value=C_T(1)
  Constant16 : Constant  Value=2
  Gain4 : Gain  Gain=Thrust_Sum  Multiplication=Matrix(K*u)
      settings: AttributesFormatString=%<Gain>
  Gain5 : Gain  Gain=C_T(2)
  Power : Math  Operator=pow  SignedPower=off  SaturateOnIntegerOverflow=on
  Product2 : Product
  Sum1 : Sum  Inputs=++|
  F_T : Outport
  wires:
  Constant15/1 -> Sum1/1
  Gain4/1 -> F_T/1  "F_T"
  n/1 -> Power/1, Gain5/1
  Power/1 -> Product2/2  "props squared"
  Gain5/1 -> Sum1/2
  Sum1/1 -> Product2/1
  Product2/1 -> Gain4/1
  Constant16/1 -> Power/2

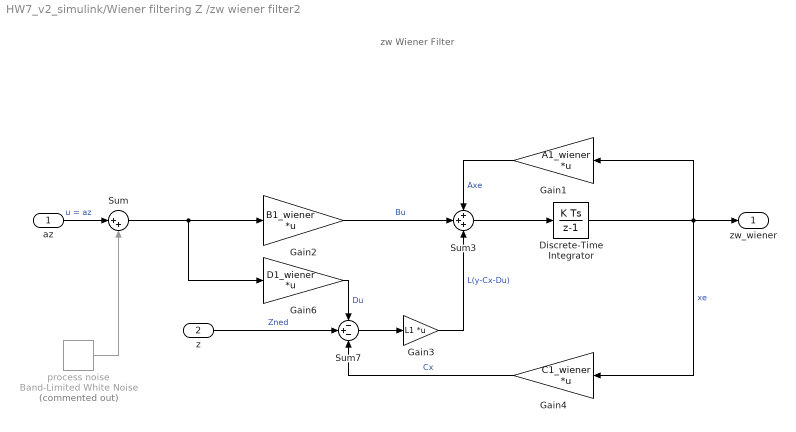
== system HW7_v2_simulink/Wiener filtering Z /zw wiener filter2 ==
  note: zw Wiener Filter
  az : Inport
  z : Inport  Port=2
  Discrete-Time Integrator : DiscreteIntegrator  SampleTime=-1  ICPrevOutput=DiscIntNeverNeededParam  ICPrevScaledInput=DiscIntNeverNeededParam
  Gain1 : Gain  Gain=A1_wiener  Multiplication=Matrix(K*u)
  Gain2 : Gain  Gain=B1_wiener  Multiplication=Matrix(K*u)
  Gain3 : Gain  Gain=L1  Multiplication=Matrix(K*u)
  Gain4 : Gain  Gain=C1_wiener  Multiplication=Matrix(K*u)
  Gain6 : Gain  Gain=D1_wiener  Multiplication=Matrix(K*u)
  Sum : Sum  Inputs=|++
  Sum3 : Sum  Inputs=+++
  Sum7 : Sum  Inputs=-+-
  process noise : simulink/Sources/Band-Limited White Noise  Commented=on  Cov=0.005  Ts=0.005  seed=[1]
  zw_wiener : Outport
  wires:
  Gain3/1 -> Sum3/3  "L(y-Cx-Du)"
  Gain1/1 -> Sum3/1  "Axe"
  Gain2/1 -> Sum3/2  "Bu"
  Discrete-Time Integrator/1 -> zw_wiener/1, Gain1/1, Gain4/1  "xe"
  Gain6/1 -> Sum7/1  "Du"
  Sum7/1 -> Gain3/1
  z/1 -> Sum7/2  "Zned"
  Gain4/1 -> Sum7/3  "Cx"
  Sum3/1 -> Discrete-Time Integrator/1
  process noise/1 -> Sum/2
  az/1 -> Sum/1  "u = az"
  Sum/1 -> Gain6/1, Gain2/1

== system HW7_v2_simulink/Wiener filtering Z 2/Zw Wiener filter ==
  note: zw Wiener Filter
  az : Inport
  z : Inport  Port=2
  Discrete-Time Integrator : DiscreteIntegrator  SampleTime=-1  ICPrevOutput=DiscIntNeverNeededParam  ICPrevScaledInput=DiscIntNeverNeededParam
  Gain1 : Gain  Gain=A1_wiener  Multiplication=Matrix(K*u)
  Gain2 : Gain  Gain=B1_wiener  Multiplication=Matrix(K*u)
  Gain3 : Gain  Gain=L1  Multiplication=Matrix(K*u)
  Gain4 : Gain  Gain=C1_wiener  Multiplication=Matrix(K*u)
  Gain6 : Gain  Gain=D1_wiener  Multiplication=Matrix(K*u)
  Sum : Sum  Inputs=|++
  Sum3 : Sum  Inputs=+++
  Sum7 : Sum  Inputs=-+-
  process noise : simulink/Sources/Band-Limited White Noise  Commented=on  Cov=0.005  Ts=0.005  seed=[1]
  zw_wiener : Outport
  wires:
  Gain3/1 -> Sum3/3  "L(y-Cx-Du)"
  Gain1/1 -> Sum3/1  "Axe"
  Gain2/1 -> Sum3/2  "Bu"
  Discrete-Time Integrator/1 -> zw_wiener/1, Gain1/1, Gain4/1  "xe"
  Gain6/1 -> Sum7/1  "Du"
  Sum7/1 -> Gain3/1
  z/1 -> Sum7/2  "Zned"
  Gain4/1 -> Sum7/3  "Cx"
  Sum3/1 -> Discrete-Time Integrator/1
  process noise/1 -> Sum/2
  az/1 -> Sum/1  "u = az"
  Sum/1 -> Gain6/1, Gain2/1

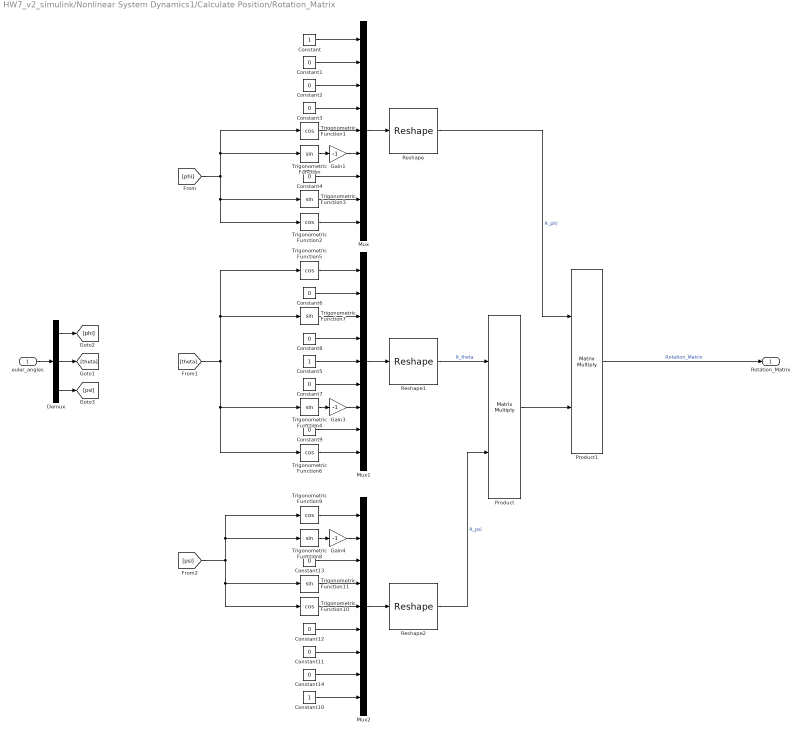
== system HW7_v2_simulink/Nonlinear System Dynamics1/Calculate Position/Rotation_Matrix ==
  "euler_angles " : Inport
  Constant : Constant
  Constant{1..4,6..9,11..14} (12 alike) : Constant  Value=0
  Constant10 : Constant
  Constant5 : Constant
  Demux : Demux  Outputs=3
  Gain1 : Gain  Gain=-1
  Gain3 : Gain  Gain=-1
  Gain4 : Gain  Gain=-1
  Mux : Mux  Inputs=9
  Mux1 : Mux  Inputs=9
  Mux2 : Mux  Inputs=9
  Product : Product  Multiplication=Matrix(*)
  Product1 : Product  Multiplication=Matrix(*)
  Reshape : Reshape  OutputDimensionality=Customize  OutputDimensions=[3,3]
  Reshape1 : Reshape  OutputDimensionality=Customize  OutputDimensions=[3,3]
  Reshape2 : Reshape  OutputDimensionality=Customize  OutputDimensions=[3,3]
  Trigonometric Function{,3..4,7..8,11} (6 alike) : Trigonometry
  Trigonometric Function{1..2,5..6,9..10} (6 alike) : Trigonometry  Operator=cos
  Rotation_Matrix : Outport
  wires:
  Constant9/1 -> Mux1/8
  Constant11/1 -> Mux2/7
  Trigonometric Function1/1 -> Mux/5
  Trigonometric Function3/1 -> Mux/8
  Constant5/1 -> Mux1/5
  Trigonometric Function7/1 -> Mux1/3
  Reshape/1 -> Product1/1  "R_phi"
  Mux1/1 -> Reshape1/1
  Trigonometric Function8/1 -> Gain4/1
  Constant7/1 -> Mux1/6
  Trigonometric Function2/1 -> Mux/9
  [phi] -> Trigonometric Function2/1, Trigonometric Function3/1, Trigonometric Function1/1, Trigonometric Function/1
  Trigonometric Function6/1 -> Mux1/9
  Constant12/1 -> Mux2/6
  Trigonometric Function4/1 -> Gain3/1
  [theta] -> Trigonometric Function7/1, Trigonometric Function5/1, Trigonometric Function4/1, Trigonometric Function6/1
  Reshape2/1 -> Product/2  "R_psi"
  Trigonometric Function/1 -> Gain1/1
  Product/1 -> Product1/2
  Trigonometric Function5/1 -> Mux1/1
  Trigonometric Function9/1 -> Mux2/1
  Mux/1 -> Reshape/1
  Constant/1 -> Mux/1
  Constant3/1 -> Mux/4
  Constant6/1 -> Mux1/2
  Mux2/1 -> Reshape2/1
  Constant2/1 -> Mux/3
  Constant1/1 -> Mux/2
  [psi] -> Trigonometric Function11/1, Trigonometric Function10/1, Trigonometric Function9/1, Trigonometric Function8/1
  Constant8/1 -> Mux1/4
  Constant4/1 -> Mux/7
  Constant13/1 -> Mux2/3
  Trigonometric Function11/1 -> Mux2/4
  Constant10/1 -> Mux2/9
  Reshape1/1 -> Product/1  "R_theta"
  Constant14/1 -> Mux2/8
  Trigonometric Function10/1 -> Mux2/5
  Product1/1 -> Rotation_Matrix/1  "Rotation_Matrix"
  Demux/3 -> [psi]
  Demux/2 -> [theta]
  "euler_angles "/1 -> Demux/1
  Demux/1 -> [phi]
  Gain3/1 -> Mux1/7
  Gain1/1 -> Mux/6
  Gain4/1 -> Mux2/2

== system HW7_v2_simulink/Nonlinear System Dynamics1/Calculate Velocity/Calculate_Thrust ==
  note: $F_{T} = \sum_{i=1}^4[0;0;C_{T}.*n.^2]$
  n : Inport
  Constant15 : Constant  Value=C_T(1)
  Constant16 : Constant  Value=2
  Gain4 : Gain  Gain=Thrust_Sum  Multiplication=Matrix(K*u)
      settings: AttributesFormatString=%<Gain>
  Gain5 : Gain  Gain=C_T(2)
  Power : Math  Operator=pow  SignedPower=off  SaturateOnIntegerOverflow=on
  Product2 : Product
  Sum1 : Sum  Inputs=++|
  F_T : Outport
  wires:
  Constant15/1 -> Sum1/1
  Gain4/1 -> F_T/1  "F_T"
  n/1 -> Power/1, Gain5/1
  Power/1 -> Product2/2  "props squared"
  Gain5/1 -> Sum1/2
  Sum1/1 -> Product2/1
  Product2/1 -> Gain4/1
  Constant16/1 -> Power/2

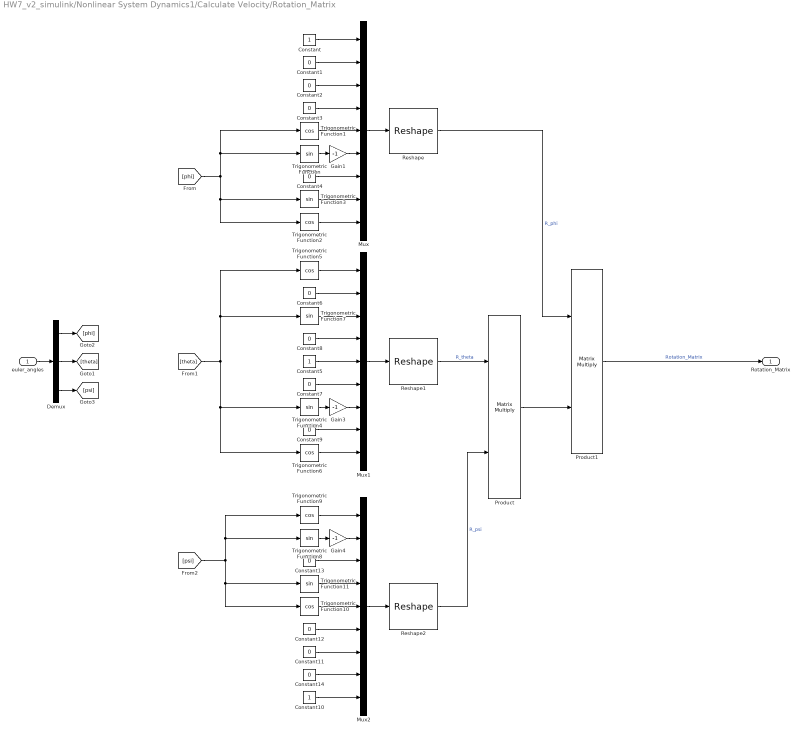
== system HW7_v2_simulink/Nonlinear System Dynamics1/Calculate Velocity/Rotation_Matrix ==
  "euler_angles " : Inport
  Constant : Constant
  Constant{1..4,6..9,11..14} (12 alike) : Constant  Value=0
  Constant10 : Constant
  Constant5 : Constant
  Demux : Demux  Outputs=3
  Gain1 : Gain  Gain=-1
  Gain3 : Gain  Gain=-1
  Gain4 : Gain  Gain=-1
  Mux : Mux  Inputs=9
  Mux1 : Mux  Inputs=9
  Mux2 : Mux  Inputs=9
  Product : Product  Multiplication=Matrix(*)
  Product1 : Product  Multiplication=Matrix(*)
  Reshape : Reshape  OutputDimensionality=Customize  OutputDimensions=[3,3]
  Reshape1 : Reshape  OutputDimensionality=Customize  OutputDimensions=[3,3]
  Reshape2 : Reshape  OutputDimensionality=Customize  OutputDimensions=[3,3]
  Trigonometric Function{,3..4,7..8,11} (6 alike) : Trigonometry
  Trigonometric Function{1..2,5..6,9..10} (6 alike) : Trigonometry  Operator=cos
  Rotation_Matrix : Outport
  wires:
  Constant9/1 -> Mux1/8
  Constant11/1 -> Mux2/7
  Trigonometric Function1/1 -> Mux/5
  Trigonometric Function3/1 -> Mux/8
  Constant5/1 -> Mux1/5
  Trigonometric Function7/1 -> Mux1/3
  Reshape/1 -> Product1/1  "R_phi"
  Mux1/1 -> Reshape1/1
  Trigonometric Function8/1 -> Gain4/1
  Constant7/1 -> Mux1/6
  Trigonometric Function2/1 -> Mux/9
  [phi] -> Trigonometric Function2/1, Trigonometric Function3/1, Trigonometric Function1/1, Trigonometric Function/1
  Trigonometric Function6/1 -> Mux1/9
  Constant12/1 -> Mux2/6
  Trigonometric Function4/1 -> Gain3/1
  [theta] -> Trigonometric Function7/1, Trigonometric Function5/1, Trigonometric Function4/1, Trigonometric Function6/1
  Reshape2/1 -> Product/2  "R_psi"
  Trigonometric Function/1 -> Gain1/1
  Product/1 -> Product1/2
  Trigonometric Function5/1 -> Mux1/1
  Trigonometric Function9/1 -> Mux2/1
  Mux/1 -> Reshape/1
  Constant/1 -> Mux/1
  Constant3/1 -> Mux/4
  Constant6/1 -> Mux1/2
  Mux2/1 -> Reshape2/1
  Constant2/1 -> Mux/3
  Constant1/1 -> Mux/2
  [psi] -> Trigonometric Function11/1, Trigonometric Function10/1, Trigonometric Function9/1, Trigonometric Function8/1
  Constant8/1 -> Mux1/4
  Constant4/1 -> Mux/7
  Constant13/1 -> Mux2/3
  Trigonometric Function11/1 -> Mux2/4
  Constant10/1 -> Mux2/9
  Reshape1/1 -> Product/1  "R_theta"
  Constant14/1 -> Mux2/8
  Trigonometric Function10/1 -> Mux2/5
  Product1/1 -> Rotation_Matrix/1  "Rotation_Matrix"
  Demux/3 -> [psi]
  Demux/2 -> [theta]
  "euler_angles "/1 -> Demux/1
  Demux/1 -> [phi]
  Gain3/1 -> Mux1/7
  Gain1/1 -> Mux/6
  Gain4/1 -> Mux2/2
